simulink model "SimulinkProject - Kopie"  (R2025b)
settings: Solver=ode5  StartTime=0.0  StopTime=100  FixedStep=0.01  RelTol=1e-3
model workspace (MAT data in the model file):
  radius = 100
settings Model: Creator=Fabian  LastModifiedBy=Fabian

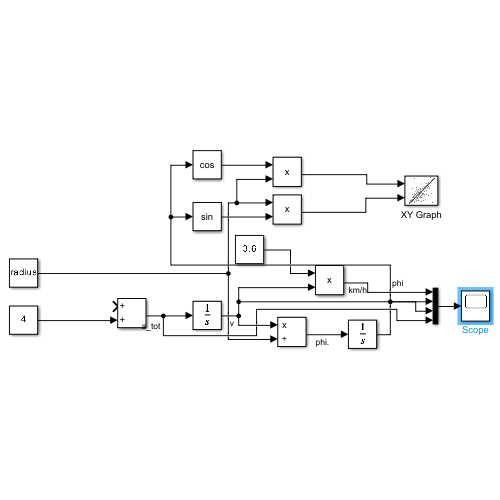
[thumbnail: Simulink's stored preview of the top-level diagram]
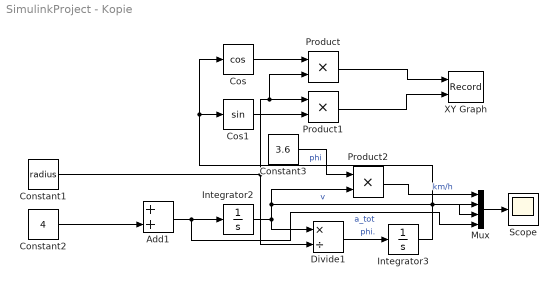
== system SimulinkProject - Kopie ==
  Add1 : Sum
  Constant1 : Constant  Value=radius
  Constant2 : Constant  Value=4
  Constant3 : Constant  Value=3.6
  Cos : Trigonometry  Operator=cos
  Cos1 : Trigonometry
  Divide1 : Product  Inputs=*/
  Integrator2 : Integrator  InitialCondition=13
  Integrator3 : Integrator  InitialCondition=pi
  Mux : Mux
  Product : Product
  Product1 : Product
  Product2 : Product
  Scope : Scope
      settings: ActiveDisplayYMinimum=-196.27602511797591  ActiveDisplayYMaximum=758.29740413414027
  XY Graph : Record  NumPorts=2.0  FileSettingsInternal="{\"entries\":[{\"content\":{\"excelSettings\":{\"content\":{},\"type\":\"Streamout.ExcelSettings\"},\"parquetSettings\":{\"content\":{},\"type\":\"Streamout.ParquetSettings\"}},\"type\":\"Streamout.FileSettingStorage\",\"uuid\":\"\"}],\"packageUris\":[\"http:\\/\\/schema.mathworks.com\\/mf0\\/streamout_blocks\\/R2020a\"],\"version\":\"1.0\"}"  FrameSettings=[0, 0]  Layout=[1 1]  SignalsInternal="{\"entries\":[{\"content\":{\"signals\":[{\"content\":{\"blockPath\":[],\"dimensions\":[1],\"domain\":\"\",\"lineColor\":\"#a2142f\",\"plots\":[ 1 ],\"port\":1,\"sid\":[\"\"],\"signalID\":1,\"signalName\":\"Product\"},\"type\":\"RecordBlkView.Signal\",\"uuid\":\"\"},{\"content\":{\"blockPath\":[],\"dimensions\":[1],\"domain\":\"\",\"lineColor\":\"#139fff\",\"plots\":[ 1 ],\"port\":2,\"sid\":[\"\"],\"signalID\":2,\"signalName\":\"Product1\"},\"type\":\"RecordBlkView.Signal\",\"uuid\":\"\"}]},\"type\":\"RecordBlkView.InputSignals\",\"uuid\":\"\"}],\"packageUris\":[\"http:\\/\\/schema.mathworks.com\\/mf0\\/streamout_blocks\\/R2020a\"],\"version\":\"1.0\"}"  VisualizationBindings="{\"xyplotplugin\":{\"info\":[{\"series\":[{\"bindingParametersList\":[{\"parameter\":\"X-Axis\",\"signalID\":1,\"signalName\":\"Product\"},{\"parameter\":\"Y-Axis\",\"signalID\":2,\"signalName\":\"Product1\"}],\"seriesID\":0}],\"subplotID\":1}]}}"  CompatibilityTag=XY
  wires:
  Add1/1 -> Mux/4, Integrator2/1  "a_tot"
  Constant1/1 -> Divide1/2, Product/2, Product1/1
  Integrator2/1 -> Product2/2, Mux/2, Divide1/1  "v"
  Divide1/1 -> Integrator3/1  "phi."
  Integrator3/1 -> Mux/3, Cos/1, Cos1/1  "phi"
  Constant2/1 -> Add1/2
  Mux/1 -> Scope/1
  Cos/1 -> Product/1
  Cos1/1 -> Product1/2
  Product/1 -> XY Graph/1
  Product1/1 -> XY Graph/2
  Product2/1 -> Mux/1  "km/h"
  Constant3/1 -> Product2/1
